simulink model "W07_PD_Noise"  (R2024b)
settings: Solver=ode45  StartTime=0.0  StopTime=t_end  MaxStep=0.001  RelTol=1e-3
PreLoadFcn:
  | % W07_PD_Noise 기본 파라미터 (모델을 열 때 자동 실행)
  | % numC, denC 는 Lead 보상기의 계수입니다.
  | defs = { 'Kp_pd',56.7 ; 'Kd_pd',18.9 ; 'r_amp',1 ; 't_end',4 ;
  |          'noise_pow',1e-8 ; 'noise_ts',0.001 ;
  |          'numG',0.01 ; 'denG',[0.005 0.06 0.1001 0] ;
  |          'numC',[265 530] ; 'denC',[1 15] };
  | for ii = 1:size(defs,1)
  |     if ~evalin('base', sprintf('exist(''%s'',''var'')', defs{ii,1}))
  |         assignin('base', defs{ii,1}, defs{ii,2});
  |     end
  | end
  | clear defs ii
values from neighbouring files (symbols this model uses):
  Kd_pd = 18.9    [W07_06_run_simulink.m]
  Kp_pd = Kd * z_pd    [W07_02_pd_and_pi.m]    (also in W07_06_run_simulink.m = 56.7)
  noise_ts = 0.001    [W07_06_run_simulink.m]
  r_amp = 1    [W07_06_run_simulink.m]
undefined symbols (not defined in the file or in its folder): denC, denG, numC, numG
libraries: simulink x1
settings Model: Creator=admin  LastModifiedBy=admin

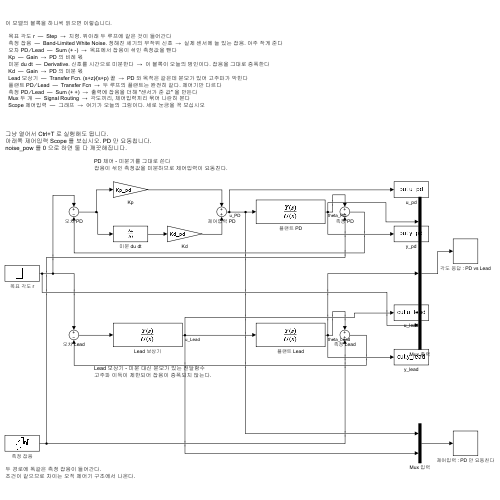
[thumbnail: Simulink's stored preview of the top-level diagram]
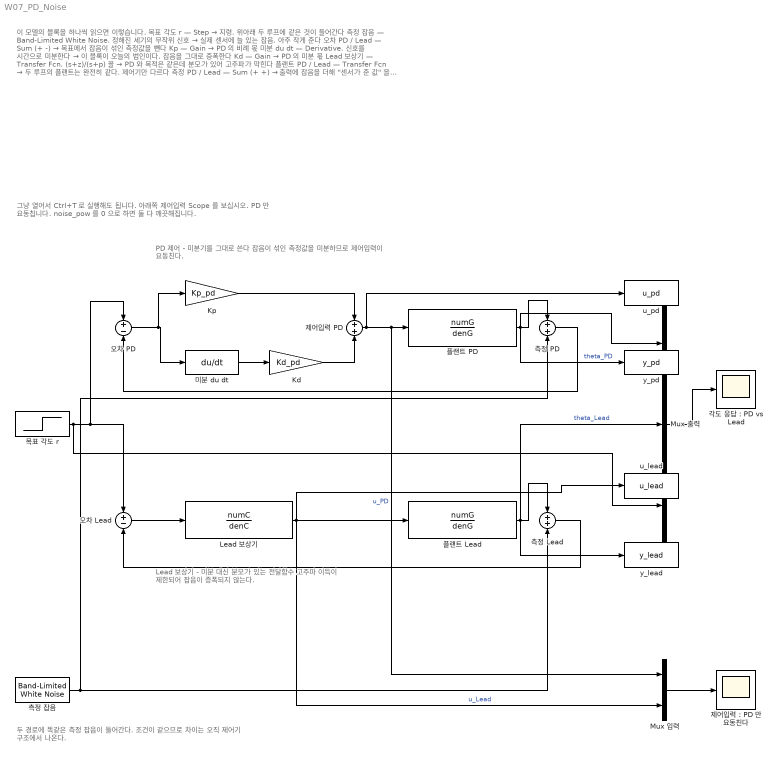
== system W07_PD_Noise ==
  note: PD 제어 - 미분기를 그대로 쓴다
      | 잡음이 섞인 측정값을 미분하므로 제어입력이 요동친다.
  note: Lead 보상기 - 미분 대신 분모가 있는 전달함수
      | 고주파 이득이 제한되어 잡음이 증폭되지 않는다.
  note: 두 경로에 똑같은 측정 잡음이 들어간다.
      | 조건이 같으므로 차이는 오직 제어기 구조에서 나온다.
  note: 그냥 열어서 Ctrl+T 로 실행해도 됩니다.
      | 아래쪽 제어입력 Scope 를 보십시오. PD 만 요동칩니다.
      | noise_pow 를 0 으로 하면 둘 다 깨끗해집니다.
  note: 이 모델의 블록을 하나씩 읽으면 이렇습니다.
      |
      |   목표 각도 r  —  Step  →  지령. 위아래 두 루프에 같은 것이 들어간다
      |   측정 잡음  —  Band-Limited White Noise. 정해진 세기의 무작위 신호  →  실제 센서에 늘 있는 잡음. 아주 작게 준다
      |   오차 PD ∕ Lead  —  Sum (+ -)  →  목표에서 잡음이 섞인 측정값을 뺀다
      |   Kp  —  Gain  →  PD 의 비례 몫
      |   미분 du dt  —  Derivative. 신호를 시간으로 미분한다  →  이 블록이 오늘의 범인이다. 잡음을 그대로 증폭한다
      |   Kd  —  Gain  →  PD 의 미분 몫
      |   Lead 보상기  —  Transfer Fcn. (s+z)∕(s+p) 꼴  →  PD 와 목적은 같은데 분모가 있어 고주파가 막힌다
      |   플랜트 PD ∕ Lead  —  Transfer Fcn  →  두 루프의 플랜트는 완전히 같다. 제어기만 다르다
      |   측정 PD ∕ Lead  —  Sum (+ +)  →  출력에 잡음을 더해 "센서가 준 값" 을 만든다
      |   Mux 두 개  —  Signal Routing  →  각도끼리, 제어입력끼리 묶어 나란히 본다
      |   Scope 제어입력  —  그래프  →  여기가 오늘의 그림이다. 세로 눈금을 꼭 보십시오
  Kd : Gain  Gain=Kd_pd
  Kp : Gain  Gain=Kp_pd
  Lead 보상기 : TransferFcn  Numerator=numC  Denominator=denC
  Mux 입력 : Mux  Inputs=2
  Mux 출력 : Mux  Inputs=3
  u_lead : ToWorkspace  VariableName=u_lead  SaveFormat=Timeseries  SampleTime=-1
  u_pd : ToWorkspace  VariableName=u_pd  SaveFormat=Timeseries  SampleTime=-1
  y_lead : ToWorkspace  VariableName=y_lead  SaveFormat=Timeseries  SampleTime=-1
  y_pd : ToWorkspace  VariableName=y_pd  SaveFormat=Timeseries  SampleTime=-1
  "각도 응답 : PD vs Lead" : Scope
  목표 각도 r : Step  Time=0  After=r_amp  SampleTime=0
  미분 du dt : Derivative
  오차 Lead : Sum  Inputs=+-
  오차 PD : Sum  Inputs=+-
  "제어입력 : PD 만 요동친다" : Scope
  제어입력 PD : Sum
  측정 Lead : Sum
  측정 PD : Sum
  측정 잡음 : simulink/Sources/Band-Limited White Noise  Cov=noise_pow  Ts=noise_ts  seed=12345
  플랜트 Lead : TransferFcn  Numerator=numG  Denominator=denG
  플랜트 PD : TransferFcn  Numerator=numG  Denominator=denG
  wires:
  목표 각도 r/1 -> 오차 PD/1, 오차 Lead/1, Mux 출력/3
  오차 PD/1 -> Kp/1, 미분 du dt/1
  미분 du dt/1 -> Kd/1
  Kp/1 -> 제어입력 PD/1
  Kd/1 -> 제어입력 PD/2
  제어입력 PD/1 -> 플랜트 PD/1, Mux 입력/1, u_pd/1  "u_PD"
  플랜트 PD/1 -> 측정 PD/1, y_pd/1, Mux 출력/1  "theta_PD"
  측정 잡음/1 -> 측정 PD/2, 측정 Lead/2
  측정 PD/1 -> 오차 PD/2
  오차 Lead/1 -> Lead 보상기/1
  Lead 보상기/1 -> 플랜트 Lead/1, u_lead/1, Mux 입력/2  "u_Lead"
  플랜트 Lead/1 -> 측정 Lead/1, y_lead/1, Mux 출력/2  "theta_Lead"
  측정 Lead/1 -> 오차 Lead/2
  Mux 출력/1 -> "각도 응답 : PD vs Lead"/1
  Mux 입력/1 -> "제어입력 : PD 만 요동친다"/1
